simulink library "AEMS_Standard_Library"  (R2016b)
settings: Solver=ode45  StartTime=0.0  StopTime=10.0  RelTol=1e-3
undefined symbols (not defined in the file or in its folder): BkPY, carto, Cbx_extegr, Cbx_lpegrsys, Cbx_portegr, Cnx_bnk_nr_conf, Cnx_cyl_nr_conf, ConfigManagement, configuration_management, Cxx_dcm_io_tmr_end_xxxx, Cxx_dcm_rt_tmr_end, Cxx_DID_xxxx_IO_max, Cxx_DID_xxxx_IO_min, Cxx_egrhsofs, Cxx_vmaniegi, DEM_DEBOUNCE_FREEZE, DEM_DTR_CTL_INVISIBLE, DEM_DTR_CTL_NORMAL, Dem_DtrId2_XXX, Dem_DtrId3_XXX, Dem_DtrId4_XXX, Dem_DtrId5_XXX, Dem_DtrId6_XXX, Dem_DtrId7_XXX, Dem_DtrId8_XXX, Dem_DtrId9_XXX, Dem_DtrId_XXX, Dem_EnableConditionId2_XXX, Dem_EnableConditionId3_XXX, Dem_EnableConditionId4_XXX, Dem_EnableConditionId5_XXX, Dem_EnableConditionId6_XXX, Dem_EnableConditionId7_XXX, Dem_EnableConditionId8_XXX, Dem_EnableConditionId_XXX, Dem_EventId, Dem_EventId2_XXX, Dem_EventId3_XXX, Dem_EventId4_XXX, Dem_EventId5_XXX, Dem_EventId6_XXX, Dem_EventId7_XXX, Dem_EventId8_XXX, Dem_EventId9_XXX, Dem_EventId_Device_Faulttype, Dem_EventId_XXX, DEM_IUMPR_GENERAL_DENOMINATOR, DEM_OPCYC_IGNITION, Dem_RatioId2_XXX, Dem_RatioId3_XXX, Dem_RatioId4_XXX, Dem_RatioId5_XXX, Dem_RatioId6_XXX, Dem_RatioId7_XXX, Dem_RatioId8_XXX, Dem_RatioId_XXX, Dem_StorageConditionId2_XXX, Dem_StorageConditionId3_XXX, Dem_StorageConditionId4_XXX, Dem_StorageConditionId5_XXX ... (+65)
libraries: AEMS_Standard_Library x477, simulink x2
(part 9 of 39)

== system AEMS_Standard_Library/LOOKUP_TABLES ==
  AEMS_DIRECTLU_1D : Subsystem  Tag=[LIB]  mask(AEMS_DIRECTLU_1D){X=Variable, BkP=BreakPoint}
      mask prompts: X "Input Variable"; BkP "BreakPoint"
      mask help:
      | This block computes one dimensional interpolation based on the given Index and Ratio
      | Please document Variable & BreakPoint parameters
      |
      | Reference to AUTOSAR specification:
      |            - AUTOSAR Service Name:  Ifl_IpoCur_f32
      |            - Reference: SWS_Ifl_00021
      mask init:
      | numDims=1;
      | interpMethod=2;
      | bp1=[-5:0.5:5];
      | tableData=atan([-5:0.5:5]);
      | if strcmp(get_param(bdroot,'BlockDiagramType'),'library')
      |   dimsChar='n';
      | else
      |   dimsChar=sprintf('%d',numDims);
      | end
      | switch interpMethod
      |   case 1
      |     plottype = 'flatplot';
      |   case 2
      |     plottype = 'lineplot';
      |   otherwise
      |     plottype = 'splineplot';
      | end
      | [x,y,xaxes,yaxes]=ndlookico(plottype,numDims,'LookupNDInterp',tableData,bp1);
      settings: AttributesFormatString=%<MaskType>\nSource Variable : %<X>\nBreakPoint : %<BkP>
      mask Help:
      | eval('path_lib=fileparts(which(''AEMS_Standard_Library''));');
      | mskblk=get_param(gcbh,'MaskType');
      | doc_path = [path_lib '\help\',mskblk,'.pdf'];
      | eval('open(doc_path)');
      mask Display:
      | text(0.5,0.75,sprintf(' %s-D T(u)',dimsChar),'horizontalAlignment','center')
      | plot(x,y)
      | plot(xaxes,yaxes)
  AEMS_DIRECTLU_2D : Subsystem  Tag=[LIB]  mask(AEMS_DIRECTLU_2D){X=Variable_X, BkPX=BreakPoint_X, Y=Variable_Y, BkPY=BreakPoint_Y}
      mask prompts: X "Input Variable X"; BkPX "BreakPoint X"; Y "Input Variable Y"; BkPY "BreakPoint Y"
      mask help:
      | This block computes the 2D interpolation based on the given index and ratio
      | Please document Variable & BreakPoint parameters
      |
      | Reference to AUTOSAR specification:
      |           - AUTOSAR Service Name:  Ifl_IpoMap_f32
      |           - Reference: SWS_Ifl_00025
      mask init:
      | numDims=2;
      | interpMethod=2;
      | bp1=[1:10];
      | tableData=peaks(10);
      | if strcmp(get_param(bdroot,'BlockDiagramType'),'library')
      |   dimsChar='n';
      | else
      |   dimsChar=sprintf('%d',numDims);
      | end
      | switch interpMethod
      |   case 1
      |     plottype = 'flatplot';
      |   case 2
      |     plottype = 'lineplot';
      |   otherwise
      |     plottype = 'splineplot';
      | end
      | [x,y,xaxes,yaxes]=ndlookico(plottype,numDims,'LookupNDInterp',tableData,bp1);
      settings: AttributesFormatString=%<MaskType>\nSource X : %<X>\nBreakPoint X : %<BkPX>\nSource Y: %<Y>\nBreakPoint Y : %<BkPY>
      mask Help:
      | eval('path_lib=fileparts(which(''AEMS_Standard_Library''));');
      | mskblk=get_param(gcbh,'MaskType');
      | doc_path = [path_lib '\help\',mskblk,'.pdf'];
      | eval('open(doc_path)');
      mask Display:
      | text(0.50,0.90,sprintf(' %s-D T(u)',dimsChar),'horizontalAlignment','center')
      | plot(x,y)
      | plot(xaxes,yaxes)
  AEMS_DIRECTLU_INDEXED_1D : Subsystem  Tag=[LIB]  mask(AEMS_DIRECTLU_INDEXED_1D){X=Variable, BkP=BreakPoint}
      mask prompts: X "Input Quantity"; BkP "BreakPoint"
      mask help:
      | Indexed interpolation 1D using Index/Ration as input
      | Please documente Variable & BreakPoint parameters
      mask init:
      | numDims=1;
      | interpMethod=1;
      | bp1=[-5:0.5:5];
      | tableData=atan([-5:0.5:5]);
      | if strcmp(get_param(bdroot,'BlockDiagramType'),'library')
      |   dimsChar='n';
      | else
      |   dimsChar=sprintf('%d',numDims);
      | end
      | switch interpMethod
      |   case 1
      |     plottype = 'flatplot';
      |   case 2
      |     plottype = 'lineplot';
      |   otherwise
      |     plottype = 'splineplot';
      | end
      | [x,y,xaxes,yaxes]=ndlookico(plottype,numDims,'LookupNDInterp',tableData,bp1);
      settings: AttributesFormatString=%<MaskType>\nSource Variable : %<X>\nBreakPoint : %<BkP>
      mask Help:
      | eval('path_lib=fileparts(which(''AEMS_Standard_Library''));');
      | doc_path = [path_lib '\help\AEMS_DIRECTLU_INDEXED_1D.pdf'];
      | eval('open(doc_path)')
      mask Display:
      | text(0.5,0.75,sprintf(' %s-D T(u)',dimsChar),'horizontalAlignment','center')
      | plot(x,y)
      | plot(xaxes,yaxes)
  AEMS_DIRECTLU_INDEXED_2D : Subsystem  Tag=[LIB]  mask(AEMS_DIRECTLU_INDEXED_2D){X=Source_X, BkPX=BreakPoint_X, Y=Source_Y, BkPY=BreakPoint_Y}
      mask prompts: X "Input Quantity X"; BkPX "BreakPoint X"; Y "Input Quantity Y"; BkPY "BreakPoint Y"
      mask help:
      | Indexed interpolation 2D using Index/Ration as inputs
      | Please documente Variable & BreakPoint parameters
      mask init:
      | numDims=2;
      | interpMethod=1;
      | bp1=[1:10];
      | tableData=peaks(10);
      | if strcmp(get_param(bdroot,'BlockDiagramType'),'library')
      |   dimsChar='n';
      | else
      |   dimsChar=sprintf('%d',numDims);
      | end
      | switch interpMethod
      |   case 1
      |     plottype = 'flatplot';
      |   case 2
      |     plottype = 'lineplot';
      |   otherwise
      |     plottype = 'splineplot';
      | end
      | [x,y,xaxes,yaxes]=ndlookico(plottype,numDims,'LookupNDInterp',tableData,bp1);
      settings: AttributesFormatString=%<MaskType>\nSource X : %<X>\nBreakPoint X : %<BkPX>\nSource Y: %<Y>\nBreakPoint Y : %<BkPY>
      mask Help:
      | eval('path_lib=fileparts(which(''AEMS_Standard_Library''));');
      | doc_path = [path_lib '\help\AEMS_DIRECTLU_INDEXED_2D.pdf'];
      | eval('open(doc_path)')
      mask Display:
      | text(0.50,0.90,sprintf(' %s-D T(u)',dimsChar),'horizontalAlignment','center')
      | plot(x,y)
      | plot(xaxes,yaxes)
  AEMS_DYNAMIC_LUT_1D : Subsystem  Tag=[LIB]  mask(AEMS_DYNAMIC_LUT_1D){}
      mask help: This block executes an interpolation in a one-dimension cartography. The input variable is automatically limited by the breakpoint table dynamics.
      mask init:
      | numDims=1;
      | interpMethod=2;
      | if strcmp(get_param(bdroot,'BlockDiagramType'),'library')
      |   dimsChar='n';
      | else
      |   dimsChar=sprintf('%d',numDims);
      | end
      | switch interpMethod
      |   case 1
      |     plottype = 'flatplot';
      |   case 2
      |     plottype = 'lineplot';
      |   otherwise
      |     plottype = 'splineplot';
      | end
      settings: AttributesFormatString=%<MaskType>
      mask Help:
      | eval('path_lib=fileparts(which(''AEMS_Standard_Library''));');
      | doc_path = [path_lib '\help\AEMS_DYNAMIC_LUT_1D.pdf'];
      | eval('open(doc_path)')
      mask Display: disp('Dynamic\n\nInterp. (1D)\n')
  AEMS_INDEXED_LUT_1D : Subsystem  Tag=[LIB]  mask(AEMS_INDEXED_LUT_1D){map_x=Cxb, map_z=Cxd}
      mask prompts: map_x "Breakpoint table :"; map_z "Lookup table (1D) :"
      mask help: This block executes a research by indexing in an one-dimension cartography. The input variable is automatically limited by the breakpoint table dynamics.
      mask init:
      | numDims=1;
      | interpMethod=1;
      | bp1=double(map_x);
      | tableData=double(map_z);
      | if strcmp(get_param(bdroot,'BlockDiagramType'),'library')
      |   dimsChar='n';
      | else
      |   dimsChar=sprintf('%d',numDims);
      | end
      | switch interpMethod
      |   case 1
      |     plottype = 'flatplot';
      |   case 2
      |     plottype = 'lineplot';
      |   otherwise
      |     plottype = 'splineplot';
      | end
      | [x,y,xaxes,yaxes]=ndlookico(plottype,numDims,'LookupNDInterp',tableData,bp1);
      settings: AttributesFormatString=%<MaskType>\nBkPX=%<map_x>\nLUT=%<map_z>
      mask Help:
      | eval('path_lib=fileparts(which(''AEMS_Standard_Library''));');
      | doc_path = [path_lib '\help\AEMS_INDEXED_LUT_1D.pdf'];
      | eval('open(doc_path)')
      mask Display:
      | text(0.5,0.75,sprintf(' %s-D T(u)',dimsChar),'horizontalAlignment','center')
      | plot(x,y)
      | plot(xaxes,yaxes)
  AEMS_INDEXED_LUT_1D_TOL : Subsystem  Tag=[LIB]  mask(AEMS_INDEXED_LUT_1D_TOL){map_x=Cxb, map_z=Cxd, Tolerance=Cxx_Tol}
      mask prompts: map_x "Breakpoint table :"; map_z "Lookup table (1D) :"
      mask help:
      | This block executes an index in a one-dimension cartography with a tolerance applied to output values of decreasing transitions between adjacent breakpoint value zones. The input variables are automatically limited  by the breakpoint tables dynamics.
      |
      | To modify the Tolerance values, right-click on the block and select "Mask Parameters...".
      mask init: same as AEMS_Standard_Library/LOOKUP_TABLES/AEMS_INDEXED_LUT_1D
      settings: AttributesFormatString=%<MaskType>\nBkPX=%<map_x>\nLUT=%<map_z>\nTolerance=%<Tolerance>
      mask Help:
      | eval('path_lib=fileparts(which(''AEMS_Standard_Library''));');
      | doc_path = [path_lib '\help\AEMS_INDEXED_LUT_1D_TOL.pdf'];
      | eval('open(doc_path)')
      mask Display:
      | text(0.50,0.90,sprintf(' %s-D T(u) with tol.',dimsChar),'horizontalAlignment','center')
      | plot(x,y)
      | plot(xaxes,yaxes)
  AEMS_INDEXED_LUT_2D : Subsystem  Tag=[LIB]  mask(AEMS_INDEXED_LUT_2D){map_x=Cxb_x, map_y=Cxb_y, carto=Cxm}
      mask prompts: map_x "X Breakpoint table :"; map_y "Y Breakpoint table :"; carto "Lookup table (2D) :"
      mask help: This block executes an index in a two-dimension cartography. The input variables are automatically limited by the breakpoint tables dynamics.
      mask init:
      | numDims=2;
      | interpMethod=1;
      | bp1=double(map_x);
      | tableData=double(carto);
      | if strcmp(get_param(bdroot,'BlockDiagramType'),'library')
      |   dimsChar='n';
      | else
      |   dimsChar=sprintf('%d',numDims);
      | end
      | switch interpMethod
      |   case 1
      |     plottype = 'flatplot';
      |   case 2
      |     plottype = 'lineplot';
      |   otherwise
      |     plottype = 'splineplot';
      | end
      | [x,y,xaxes,yaxes]=ndlookico(plottype,numDims,'LookupNDInterp',tableData,bp1);
      settings: AttributesFormatString=%<MaskType>\nBkPX=%<map_x>\nBkPY=%<map_y>\nMAP=%<carto>
      mask Help:
      | eval('path_lib=fileparts(which(''AEMS_Standard_Library''));');
      | doc_path = [path_lib '\help\AEMS_INDEXED_LUT_2D.pdf'];
      | eval('open(doc_path)')
      mask Display:
      | text(0.50,0.90,sprintf(' %s-D T(u)',dimsChar),'horizontalAlignment','center')
      | plot(x,y)
      | plot(xaxes,yaxes)
  AEMS_INDEXED_LUT_2D_TOL : Subsystem  Tag=[LIB]  mask(AEMS_INDEXED_LUT_2D_TOL){map_x=Cxb_X, map_y=Cxb_Y, carto=Cxm, X_Tolerance=Cxx_Tol_X, Y_Tolerance=Cxx_Tol_Y}
      mask prompts: map_x "X Breakpoint table :"; map_y "Y Breakpoint table :"; carto "Lookup table (2D) :"
      mask help:
      | This block executes an index in a two-dimension cartography with a tolerance applied to output values of decreasing transitions between adjacent breakpoint value zones. The input variables are automatically limited  by the breakpoint tables dynamics.
      |
      | To modify the Tolerance values, right-click on the block and select "Mask Parameters...".
      mask init: same as AEMS_Standard_Library/LOOKUP_TABLES/AEMS_INDEXED_LUT_2D
      settings: AttributesFormatString=%<MaskType>\nBkPX=%<map_x>\nBkPY=%<map_y>\nMAP=%<carto>\nToleranceX=%<X_Tolerance>\nToleranceY=%<Y_Tolerance>
      mask Help:
      | eval('path_lib=fileparts(which(''AEMS_Standard_Library''));');
      | doc_path = [path_lib '\help\AEMS_INDEXED_LUT_2D_TOL.pdf'];
      | eval('open(doc_path)')
      mask Display:
      | text(0.50,0.90,sprintf(' %s-D T(u) with tol.',dimsChar),'horizontalAlignment','center')
      | plot(x,y)
      | plot(xaxes,yaxes)
  AEMS_INTERP : Subsystem  Tag=[LIB]  Description=This library calculates interpolation for 2 inputs.  mask(AEMS_INTERP){}
      mask help:
      | Interpolation for 2inputs
      |
      | output = input_of_ratio_1 * interpolate_ratio
      |          + input_of_ratio_0 * ( 1 - interpolate_ratio )
      |
      | I/O
      |     input_of_ratio_1
      |         Input of ratio term
      |     input_of_ratio_0
      |         Input of 1 - ratio term
      |     interpolate_ratio
      |         Interpolate Ratio ( 0 <= interpolate_ratio <= 1 )
      |
      |     output
      |         Output value
      settings: AttributesFormatString=%<MaskType>
      mask Help:
      | eval('path_lib=fileparts(which(''AEMS_Standard_Library''));');
      | mskblk=get_param(gcbh,'MaskType');
      | doc_path = [path_lib '\help\',mskblk,'.pdf'];
      | eval('open(doc_path)');
  AEMS_ITP3D : Subsystem  Tag=[LIB]  mask(AEMS_ITP3D){}
      mask help:
      | Vxx_fac is the parameter to interpolate between the three inputs
      |
      | The variable Vxx_fac is limited between 1 and 3.
      | If Vxx_fac == 1,  then Vxx_output == Vxx_in1
      | If Vxx_fac == 2,  then Vxx_output == Vxx_in2
      | If Vxx_fac == 3 , then Vxx_output == Vxx_in3
      |
      | If the Vxx_fac is not an integer, then Vxx_out is the result of interpolation.
      settings: AttributesFormatString=%<MaskType>
      mask Help:
      | eval('path_lib=fileparts(which(''AEMS_Standard_Library''));');
      | doc_path = [path_lib '\help\AEMS_ITP3D.pdf'];
      | eval('open(doc_path)')
      mask Display: disp('AEMS_ITP3D');
  AEMS_LUT_1D : Subsystem  Tag=[LIB]  mask(AEMS_LUT_1D){map_x=Cxb, map_z=Cxp}
      mask prompts: map_x "Breakpoint array :"; map_z "Lookup table (1D) :"
      mask help:
      | This block executes an interpolation in one-dimensional cartography. The input variable is automatically limited  by the breakpoint table dynamics.
      |
      | Reference to AUTOSAR specification:
      |            - AUTOSAR Service Name:  Ifl_IntIpoCur_f32_f32
      |            - Reference: SWS_Ifl_00035
      mask init:
      | numDims=1;
      | interpMethod=2;
      | bp1=double(map_x);
      | tableData=double(map_z);
      | if strcmp(get_param(bdroot,'BlockDiagramType'),'library')
      |   dimsChar='n';
      | else
      |   dimsChar=sprintf('%d',numDims);
      | end
      | switch interpMethod
      |   case 1
      |     plottype = 'flatplot';
      |   case 2
      |     plottype = 'lineplot';
      |   otherwise
      |     plottype = 'splineplot';
      | end
      | [x,y,xaxes,yaxes]=ndlookico(plottype,numDims,'LookupNDInterp',tableData,bp1);
      settings: AttributesFormatString=%<MaskType>\nBkPX=%<map_x>\nLUT=%<map_z>
      mask Help:
      | eval('path_lib=fileparts(which(''AEMS_Standard_Library''));');
      | mskblk=get_param(gcbh,'MaskType');
      | doc_path = [path_lib '\help\',mskblk,'.pdf'];
      | eval('open(doc_path)');
      mask Display:
      | text(0.5,0.75,sprintf(' %s-D T(u)',dimsChar),'horizontalAlignment','center')
      | plot(x,y)
      | plot(xaxes,yaxes)
  AEMS_LUT_2D : Subsystem  Tag=[LIB]  mask(AEMS_LUT_2D){map_x=Cxb_x, map_y=Cxb_y, carto=Cxm}
      mask prompts: map_x "X Breakpoint array :"; map_y "Y Breakpoint array :"; carto "Lookup table (2D) :"
      mask help:
      | This block executes an interpolation in two-dimensional cartography. The input variables are automatically limited  by the breakpoint tables dynamics.
      |
      | Reference to AUTOSAR specification:
      |            - AUTOSAR Service Name:  Ifl_IntIpoMap_f32f32_f32
      |            - Reference: SWS_Ifl_00041
      mask init:
      | numDims=2;
      | interpMethod=2;
      | bp1=double(map_x);
      | tableData=double(carto);
      | if strcmp(get_param(bdroot,'BlockDiagramType'),'library')
      |   dimsChar='n';
      | else
      |   dimsChar=sprintf('%d',numDims);
      | end
      | switch interpMethod
      |   case 1
      |     plottype = 'flatplot';
      |   case 2
      |     plottype = 'lineplot';
      |   otherwise
      |     plottype = 'splineplot';
      | end
      | [x,y,xaxes,yaxes]=ndlookico(plottype,numDims,'LookupNDInterp',tableData,bp1);
      settings: AttributesFormatString=%<MaskType>\nBkPX=%<map_x>\nBkPY=%<map_y>\nMAP=%<carto>
      mask Help:
      | eval('path_lib=fileparts(which(''AEMS_Standard_Library''));');
      | mskblk=get_param(gcbh,'MaskType');
      | doc_path = [path_lib '\help\',mskblk,'.pdf'];
      | eval('open(doc_path)');
      mask Display:
      | text(0.50,0.90,sprintf(' %s-D T(u)',dimsChar),'horizontalAlignment','center')
      | plot(x,y)
      | plot(xaxes,yaxes)
  AEMS_PRE_INTERP : Subsystem  Tag=[LIB]  mask(AEMS_PRE_INTERP){Cxb=Breakpoint}
      mask prompts: Cxb "BreakPoint array"
      mask help:
      | The block computes the Index and Ratio of input variable in a breakpoint data
      |
      | Reference to AUTOSAR specification:
      |            - AUTOSAR Service Name:  Ifl_DPSearch_f32
      |            - Reference: SWS_Ifl_00010
      mask init:
      | fig='f';
      | f='f';
      | [x,y]=ndlookico('bpplotdata',fig);
      | [xp,yp]=ndlookico('bppatchdata');
      settings: AttributesFormatString=%<MaskType>\nBKPT = %<Cxb>
      mask Help:
      | eval('path_lib=fileparts(which(''AEMS_Standard_Library''));');
      | mskblk=get_param(gcbh,'MaskType');
      | doc_path = [path_lib '\help\',mskblk,'.pdf'];
      | eval('open(doc_path)');
      mask Display:
      | text(2.3*0.13, .95*0.85, '','HorizontalAlignment','center','VerticalAlignment','middle');
      | text(0.4, 0.53, '','HorizontalAlignment','center','VerticalAlignment','base');
      | text(0.88, 0.3, '','HorizontalAlignment','center','VerticalAlignment','middle');
      | plot(0.3+0.4*x,0.4+0.3*y);
      | patch(0.3+0.4*xp, 0.4+0.3*yp);

== system AEMS_Standard_Library/MATH ==
  AEMS_CLAMP : Subsystem  Tag=[LIB]  mask(AEMS_CLAMP){}
      mask help:
      | This block returns the bounded value (Output), determined according to the following equation
      |
      | Output = Min, if Input ≤ Min
      | Output = Max, if Input ≥ Max
      | Output = Input, if Min < val < Max
      |
      | Reference to AUTOSAR specification:
      |          - AUTOSAR Service Name:  Mfl_Limit_f32
      |          - Reference: SWS_Mfl_00122
      settings: AttributesFormatString=%<MaskType>
      mask Help:
      | eval('path_lib=fileparts(which(''AEMS_Standard_Library''));');
      | mskblk=get_param(gcbh,'MaskType');
      | doc_path = [path_lib '\help\',mskblk,'.pdf'];
      | eval('open(doc_path)');
      mask Display: plot([0.2 0.8],[0.5 0.5],[0.5 0.5],[0.2 0.8],[0.2 0.35 0.65 0.8],[0.2 0.2 0.8 0.8])
  AEMS_DIVISION_BY_ZERO : Subsystem  Tag=[LIB]  mask(AEMS_DIVISION_BY_ZERO){Tolerence=1.1920929e-07}
      mask prompts: Tolerence "Denominator Tolerance"
      mask help:
      | This block outputs the value of the division operation "num / den ". If the "den" is exactly 0,the output will be the value at the port "ans_of_0div"
      |
      | In order to avoid "Inf" at output ,"den" must not take values close to zero.
      | Please provide Denominator tolerance(lowest possible resolution that denominator can take) in the mask.
      | Default tolerance: 1.1920929e-07
      mask init:
      | if Tolerence < 0
      |     errordlg('Denominator Tolerance value must be positive', 'Error Message');
      | end
      settings: AttributesFormatString=%<MaskType>\nDenominator Tolerance = %<Tolerence>
      mask Help:
      | eval('path_lib=fileparts(which(''AEMS_Standard_Library''));');
      | doc_path = [path_lib '\help\AEMS_DIVISION_BY_ZERO.pdf'];
      | eval('open(doc_path)')
      mask Display:
      | port_label('input',1,'den')
      | port_label('input',2,'num')
      | port_label('output',1,'result')
      | port_label('input',3,'ans_of_0div')
      | disp('Division \n no division by "0"')
      | 
      | disp('\n\n\n\n!! This Block is obsolete and should be replaced \n by AEMS_PROTECTED_DIVISION instead')
  AEMS_EXTRACT_INDEX : Subsystem  Tag=[LIB]  mask(AEMS_EXTRACT_INDEX){}
      mask help:
      | This block is built to extract the previous value (Previous_Value) and the corresponding index (Index_prev) as well as the next value (Next_Value) and its corresponding index (Index_nxt) of an increasing vector when compared to a scalar input (X).
      |
      | If the scalar input is smaller than all elements of Vector. The previous index is the smallest index, the next index is equal to previous index plus 1.
      |
      | If the scalar input is greater than all elements of Vector, the previous value and the next value are the same; it is the last value of the vector. The previous index and the next have the greatest index.
      settings: AttributesFormatString=%<MaskType>
      mask Help:
      | eval('path_lib=fileparts(which(''AEMS_Standard_Library''));');
      | doc_path = [path_lib '\help\AEMS_EXTRACT_INDEX.pdf'];
      | eval('open(doc_path)')
  AEMS_IGN_TO_PHY : Subsystem  Tag=[LIB]  mask(AEMS_IGN_TO_PHY){nb_cyl_max=6}
      mask prompts: nb_cyl_max "Limitation of number of cylinders"
      mask help:
      | Converts a vector that is supposed to be an ignition order into cylinder physical order given by the "order vector" calibration input.
      | Number of cylinders can be handled is from 1 cylinder to 6 cylinders. Calibration should indicate 0 when cylinders are not used.
      | Limitation of number of cylinders : the number of cylinders really used in input/output.
      | If some elements of the vectors are not used, a replacement value is asked as an input of the block.
      |
      | -INPUTS-
      | Order_vector: Order to sort
      | Replacement value: Value to be replaced for unused index
      | Ignition order:Physical order: Vector to be sorted
      |
      | -OUTPUTS-
      | Physical order: Ouput vector sorted
      |
      | -PARAMETERS-
      | Limitation of number of cylinders: Limit of cylinder number
      mask init:
      | Input='Ignition order';
      | Output='Physical order';
      settings: AttributesFormatString=%<MaskType>\nLimitation of number of cylinders = %<nb_cyl_max>
      mask Help:
      | eval('path_lib=fileparts(which(''AEMS_Standard_Library''));');
      | doc_path = [path_lib '\help\AEMS_IGN_TO_PHY.pdf'];
      | eval('open(doc_path)')
      mask Display:
      | port_label('input',1,'Order vector');
      | port_label('input',2,'Replacement value');
      | port_label('input',3,Input);
      | port_label('output',1,Output);
  AEMS_MATRIX_INVERSION : Subsystem  Tag=[LIB]  mask(AEMS_MATRIX_INVERSION){}
      mask help:
      | Computes the inversion of a 3*3 matrix.
      |
      | Input: Must be a 3*3 matrix.
      | Output: Inverse of the given input 3*3 matrix.
      |
      | For Example, If Matrix A (3*3 dimension), then the inverse is computed by, Inverse A = (1/Det(A)*Adj(A)).
      |
      | Note: If the Det(A) =0, then matrix inversion is not possible.
      | So, the output will be the alternate input.
      settings: AttributesFormatString=%<MaskType>
      mask Help:
      | eval('path_lib=fileparts(which(''AEMS_Standard_Library''));');
      | doc_path = [path_lib '\help\AEMS_MATRIX_INVERSION.pdf'];
      | eval('open(doc_path)')
      mask Display:
      | disp('\n\n\n\n\n\nAEMS_MATRIX_INVERSION')
      | plot([0.32 0.32],[0.3 0.9],[0.62 0.62],[0.3 0.9])
      | text(0.35,0.8,'x1');
      | text(0.45,0.8,'x2');
      | text(0.55,0.8,'x3');
      | text(0.35,0.6,'y1');
      | text(0.45,0.6,'y2');
      | text(0.55,0.6,'y3');
      | text(0.35,0.4,'z1');
      | text(0.45,0.4,'z2');
      | text(0.55,0.4,'z3');
      | plot([0.32 0.35],[0.3 0.3])
      | plot([0.59 0.62],[0.3 0.3])
      | plot([0.32 0.35],[0.9 0.9])
      | plot([0.59 0.62],[0.9 0.9])
      | plot([0.65 0.67],[0.92 0.92])
      | %plot([0.70 0.70],[0.85 1])
      | text(0.68,0.9,'1')
  AEMS_PHY_TO_IGN : Subsystem  Tag=[LIB]  mask(AEMS_PHY_TO_IGN){nb_cyl_max=6}
      mask prompts: nb_cyl_max "Limitation of number of cylinders"
      mask help:
      | Converts a vector that is supposed to be in Cylinder Physical order to an ignition order given by the "Order vector" calibration input (always of dimension 1x6).
      | Number of cylindres can be handled is from 1 cylinder to 6 cylinders.
      | Calibration should indicate 0 when cylinders are not used.
      |
      | Limitation of number of cylinders : the number of cylinders really used in input/output.
      |
      | If some elements of the vectors are not used, a replacement value is asked as an input of the block.
      mask init:
      | Output='Ignition order';
      | Input='Physical order';
      settings: AttributesFormatString=%<MaskType>\nLimitation of number of cylinders = %<nb_cyl_max>
      mask Help:
      | eval('path_lib=fileparts(which(''AEMS_Standard_Library''));');
      | doc_path = [path_lib '\help\AEMS_PHY_TO_IGN.pdf'];
      | eval('open(doc_path)')
      mask Display:
      | port_label('input',1,'Order vector');
      | port_label('input',2,'Replacement value');
      | port_label('input',3,Input);
      | port_label('output',1,Output);
  AEMS_PROTECTED_DIVISION : Subsystem  Tag=[LIB]  mask(AEMS_PROTECTED_DIVISION){out_mode=Numerator / Tolerance -> Output, tolerance=0.01}
      mask prompts: out_mode "Output when |Denominator| < Tolerance"; tolerance "Denominator Tolerance"
      mask help:
      | This block outputs the value of the division operation "num / den".
      | When the "den" is less than "Denominator Tolerance", then there are two possible outputs that can be chosen:
      | Case 1: The output will be the value at the port "default_output".
      | Case 2: The output will be "Numerator/Tolerance".
      |
      | Note :
      | For TargetLink Code generation, "protect against division by zero in production code" property should be disabled for the divide block present inside this Library.
      |
      | The "tolerance" value has to be given in accordance with the "den" (denominator) datatype.
      mask init:
      | This_Blk=gcb;
      | if tolerance < 0
      |     errordlg('Denominator tolerance value must be positive', 'Error Message');
      | end
      | 
      | ports = get_param(gcb,'PortHandles');
      | nbinport = length(ports.Inport);
      | 
      | if(out_mode == 1) %default ouput, three inputs
      |     if(nbinport==2)%change things => three inputs
      |     delete_line(This_Blk,'Divide/1','result/1');
      |     add_block('built-in/Inport',[This_Blk,'/default_output'],'Position',[85   448   105   462],'BackgroundColor','Green');
      |     add_block('simulink/Signal Routing/Switch',[This_Blk,'/Switch1'],'Position',[695   293   735   487],'Criteria','u2 ~= 0',...
      |          'AttributesFormatString','Criteria=%<Criteria>','ShowName','off');
      |     add_line(This_Blk,'Divide/1','Switch1/1','autorouting','on');
      |     add_line(This_Blk,'RelationalOperator/1','Switch1/2','autorouting','on');
      |     add_line(This_Blk,'default_output/1','Switch1/3','autorouting','on');
      |     add_line(This_Blk,'Switch1/1','result/1','autorouting','on');
      |     end
      |     ModeStr = 'Default_Output -> Output';
      |     
      | elseif(out_mode == 2) % tol used as denominator, two inputs
      |     if(nbinport==3)%change things => two inputs
      |     delete_block([This_Blk,'/default_output']);
      |     delete_block([This_Blk,'/Switch1']);
      |     delete_line(find_system(This_Blk,'FindAll','on','FollowLinks','on','LookUnderMasks','on','Type','line','Connected','off')); 
      |     add_line(This_Blk,'Divide/1','result/1');
      |     end
      |     ModeStr = 'Numerator / Tolerance -> Output';
      | end
      settings: AttributesFormatString=%<MaskType>\nOutput when |Denominator| < Tolerance = %<out_mode>\nDenominator Tolerance = %<tolerance>
      mask Help:
      | eval('path_lib=fileparts(which(''AEMS_Standard_Library''));');
      | mskblk=get_param(gcbh,'MaskType');
      | doc_path = [path_lib '\help\',mskblk,'.pdf'];
      | eval('open(doc_path)');
      mask TypeOptions out_mode: Default_Output -> Output | Numerator / Tolerance -> Output
      mask Display: disp(['Protected division\n' ModeStr])
  AEMS_SORT : Subsystem  Tag=[LIB]  TreatAsAtomicUnit=on  mask(AEMS_SORT){N=20, SortChoice=Ascendant Median, IndexSelection=on}
      mask prompts: N "Number of input element"; SortChoice "Way of sorting"; IndexSelection "Selectable Index"
      mask help:
      | This block is used to sort one-dimensional arrays and to get the median in the case of the ascending sorting.
      |
      | You have the choice between 3 options which are :
      | - Option 1 : Sort in ascending order
      | - Option 2 : Sort in descending order
      | - Option 3 : Sort in ascending order and get the corresponding median
      |
      | In addition, you can choose or not to select the number of element that you want to sort in your table and get the median number with the Option 3. (This input number N is the desired size of the input matrix that you want to sort, from 0 to N index ).
      |
      | - INPUTS -
      |
      | If the "selectable index" option is checked
      | - Disordered 1-D vector
      | - The first N numbers that you want to sort (zero-based index)
      |
      | If the "selectable index" option is unchecked :
      | - Disordered 1-D vector
      |
      | - OUTPUTS -
      |
      | =>For the Option 1&2
      | - If the check box "selectable index" is checked : Sorted vector of the first N numbers
      | - If the checkbox "selectable index" is not checked : Sorted vector of  the whole matrix
      |
      | =>For the Option 3
      | - If the checkbox "selectable index" is checked : Sorted vector and median of the first N numbers
      | - If the checkbox "selectable index" is not checked : Sorted vector and median of  the whole matrix
      |
      | NOTE: The maximum value allowed for the input "Selectable index" is 127.
      mask init:
      | block = find_system(gcb,...
      |           'LookUnderMasks','on',...
      |           'FollowLinks','on','Name','Median_Out');
      | 
      | %%%%%%%%%%%%%%
      | 
      | %condition for the selectable index
      | 
      | if strcmpi(IndexSelection,'on')
      |     
      |     if ismember(get_param([gcb, '/Index'],'BlockType'),{'Inport'})   
      |     else
      |      replace_block(gcb,'FollowLinks','on','Name','Index','built-in/Inport','noprompt');
      |      set_param([gcb, '/Index'],'BackgroundColor','green')
      |     end
      | 
      | else
      |    replace_block(gcb,'FollowLinks','on','Name','Index','Constant','noprompt');
      |    set_param([gcb, '/Index'], 'Value', 'N-1','OutDataTypeStr','uint8');
      | end
      | 
      | %%%%%%%%%%%%%%
      | 
      | set_param([gcb, '/For_loop_1/For_loop_2/Comparison/Selector'], 'InputPortWidth', 'N')
      | set_param([gcb, '/For_loop_1/For_loop_2/Comparison/Selector1'], 'InputPortWidth', 'N')
      | set_param([gcb, '/For_loop_1/For_loop_2/UnitDelay'], 'InitialCondition', 'zeros(1,N)')
      | 
      | switch SortChoice
      |     case 1
      |         set_param([gcb,'/For_loop_1/For_loop_2/Comparison/Relational_Operator'], 'Operator', '>')
      |         if ~isempty(block)
      |             delete_line([gcb],'For_loop_1/1','AEMS_SORT_MEDIAN/1')
      |             delete_line([gcb],'Index/1','AEMS_SORT_MEDIAN/2')
      |             delete_line([gcb],'AEMS_SORT_MEDIAN/1','Median_Out/1')
      |             delete_block([gcb,'/AEMS_SORT_MEDIAN'])
      |             delete_block(block);
      |         end
      |             
      |             
      |     case 2
      |         set_param([gcb, '/For_loop_1/For_loop_2/Comparison/Relational_Operator'], 'Operator', '<')
      |         if ~isempty(block)
      |             delete_line([gcb],'For_loop_1/1','AEMS_SORT_MEDIAN/1')
      |             delete_line([gcb],'Index/1','AEMS_SORT_MEDIAN/2')
      |             delete_line([gcb],'AEMS_SORT_MEDIAN/1','Median_Out/1')
      |             delete_block([gcb,'/AEMS_SORT_MEDIAN'])
      |             delete_block(block);
      |         end
      |             
      | 
      |     case 3 
      |         set_param([gcb, '/For_loop_1/For_loop_2/Comparison/Relational_Operator'], 'Operator', '>')
      |         if isempty(block)
      |             add_block('built-in/Outport',[gcb,'/Median_Out'],'Position',[815 178 845 192],'BackgroundColor','Orange');
      |             add_block('AEMS_Standard_Library/SUB/AEMS_SORT_MEDIAN',[gcb,'/AEMS_SORT_MEDIAN'],'Position',[525 139 720 226]);
      |             add_line([gcb],{'For_loop_1/1','Index/1'},{'AEMS_SORT_MEDIAN/1','AEMS_SORT_MEDIAN/2'},'autorouting','on')
      |             add_line([gcb],'AEMS_SORT_MEDIAN/1','Median_Out/1','autorouting','on')
      |         end
      |  end
      settings: AttributesFormatString=%<MaskType>\nSize of input vector : %<N>\n Sort : %<SortChoice>\nSelectable Index = %<IndexSelection>
      mask Help:
      | eval('path_lib=fileparts(which(''AEMS_Standard_Library''));');
      | doc_path = [path_lib '\help\AEMS_SORT.pdf'];
      | eval('open(doc_path)')
      mask TypeOptions SortChoice: Ascendant | Descendant | Ascendant Median
      mask Display:
      | set_param(gcb,'BackgroundColor','yellow');
      | 
      | text(0.40,0.1,'AEMS_SORT');
      | 
      | %upper box
      | plot([0.3 0.35],[0.7 0.7], [0.3 0.35],[0.65 0.65], [0.3 0.3],[0.7 0.65], [0.35 0.35],[0.7 0.65])
      | plot([0.4 0.45],[0.7 0.7], [0.4 0.45],[0.65 0.65], [0.4 0.4],[0.7 0.65], [0.45 0.45],[0.7 0.65])
      | plot([0.5 0.55],[0.7 0.7], [0.5 0.55],[0.65 0.65], [0.5 0.5],[0.7 0.65], [0.55 0.55],[0.7 0.65])
      | plot([0.6 0.65],[0.7 0.7], [0.6 0.65],[0.65 0.65], [0.6 0.6],[0.7 0.65], [0.65 0.65],[0.7 0.65])
      | 
      | %lower box
      | plot([0.3 0.35],[0.35 0.35], [0.3 0.35],[0.3 0.3], [0.3 0.3],[0.3 0.35], [0.35 0.35],[0.3 0.35])
      | plot([0.4 0.45],[0.35 0.35], [0.4 0.45],[0.3 0.3], [0.4 0.4],[0.3 0.35], [0.45 0.45],[0.3 0.35])
      | 
      | %boxes
      | plot([0.5 0.55],[0.35 0.35], [0.5 0.55],[0.3 0.3], [0.5 0.5],[0.3 0.35], [0.55 0.55],[0.3 0.35])
      | plot([0.6 0.65],[0.35 0.35], [0.6 0.65],[0.3 0.3], [0.6 0.6],[0.3 0.35], [0.65 0.65],[0.3 0.35])
      | 
      | %lines
      | plot([0.32 0.62],[0.65 0.35], [0.62 0.42],[0.65 0.35], [0.42 0.32],[0.65 0.35], [0.52 0.52],[0.65 0.35])
      | 
      | %arrows
      | plot([0.32 0.32],[0.35 0.43], [0.32 0.36],[0.35 0.39])
      | plot([0.42 0.44],[0.35 0.43], [0.42 0.465],[0.35 0.37])
      | plot([0.52 0.5],[0.35 0.41], [0.52 0.54],[0.35 0.4])
      | plot([0.62 0.6],[0.35 0.4], [0.62 0.58],[0.35 0.36])
      | 
      | port_label('input',1,'Vector to sort');
      | 
      | port_label('output',1,'Sorted vector 0:N');
      | 
      | switch SortChoice
      | 
      |     case 3
      |         port_label('output',2,'Median vector 0:N');
      | end
      | 
      | 
      | if strcmpi(IndexSelection,'on')
      |     port_label('input',2,'Selectable index 0:N');
      | end
  AEMS_SQRT : Subsystem  Tag=[LIB]  mask(AEMS_SQRT){FunctionOfSqrt=signedSqrt}
      mask prompts: FunctionOfSqrt "Function of Sqrt"
      mask help:
      | This block returns the square root of the input. (signedSqrt / rSqrt)
      | It can perform square root operation for both signed and unsigned values. But according to AUTOSAR service Mfl_Sqrt_f32 only unsigned inputs are allowed.
      |
      | Reference to AUTOSAR specification:
      | - AUTOSAR Service Name:  Mfl_Sqrt_f32 (Ref. [SWS_Mfl_00135])
      |
      | Function of Sqrt:
      | <signedSqrt>: Square root of the absolute value of the input, multiplied by the sign of the input
      | <rSqrt>: Reciprocal of square root of the input
      mask init:
      | This_Blk=gcb;
      | Bpath = [This_Blk,'/Sqrt'];
      | FunctionOfSqrt = get_param(This_Blk,'FunctionOfSqrt');
      | set_param(Bpath,'Operator',FunctionOfSqrt);
      settings: AttributesFormatString=|
      | %<MaskType> \n Service name : Mfl_Sqrt_f32
      | Function of Sqrt  : %<FunctionOfSqrt>
      mask Help:
      | eval('path_lib=fileparts(which(''AEMS_Standard_Library''));');
      | mskblk=get_param(gcbh,'MaskType');
      | doc_path = [path_lib '\Help\',mskblk,'.pdf'];
      | eval('open(doc_path)');
      mask TypeOptions FunctionOfSqrt: signedSqrt | rSqrt
      mask Display: disp('AEMS_SQRT\n');

== system AEMS_Standard_Library/MEM ==
  AEMS_NVM_SET : UnitDelay  Tag=[LIB]  InitialCondition=initial_value  SampleTime=-1  mask(AEMS_NVM_SET){initial_value=0}
      mask help: 'Unit Delay' for NVM(non volatile memory).
      settings: AttributesFormatString=<initial=%<initial_value>>
      mask Display:
      | % patch([0 100 100 0], [100 100 0 0], [1 1 1])
      | 
      | text(50,50,'\fontsize{14}1/Z','HorizontalAlignment','center',...
      |     'VerticalAlignment','middle','texmode','on')
      | text(92,100,'\fontsize{10}NVM ','HorizontalAlignment','right',...
      |     'VerticalAlignment','top','texmode','on')
      | 
      | plot([0,100],[0,0])
      | plot([0,100],[100,100])
      | plot([0,0],[0,100])
      | plot([100,100],[0,100])
  AEMS_NVM_WRITEONFLY : Subsystem  Tag=[LIB]  mask(AEMS_NVM_WRITEONFLY){NumInputs=1, ChId=<AEMS_Specification_Name>, TriggerType=Rising edge}
      mask prompts: NumInputs "Number of Inputs"; ChId "Channel Name (AEMS Specification Name):"; TriggerType "Trigger Type"
      mask help:
      | This block allows to represent the NVM write ON FLY Storage Type which will generate during codegeneration process (example):
      |
      | if (NVM_trigger && !NVMtrigger_old )
      |        Event_WriteOnFly_<AEMS_Specification_Name>();
      | end
      |
      | The parameter TriggerType can either be Rising edge (default) or Enable.
      |
      | NOTE: Input must not be zero.
      mask init:
      | % AEMSPattern='^[a,b]_...._...._..._\w*';
      | % if isempty(regexp(ChId,AEMSPattern,'once'))
      | %    errordlg('Error! Channel name is not correct');
      | % end
      | ThisBlk=gcb;
      | BlkType_Of_TriggerType  = get_param([ThisBlk '/PortType'] ,'BlockType');
      | TriggerType=get_param(ThisBlk,'TriggerType');
      | if isequal(TriggerType,'Rising edge')
      |     if strcmp(BlkType_Of_TriggerType ,'TriggerPort')
      |     %do nothing
      |     else
      |     replace_block(ThisBlk,'FollowLinks','on','Name','PortType','simulink/Ports & Subsystems/Trigger','noprompt');
      |     end
      | else
      |     if strcmp(BlkType_Of_TriggerType ,'EnablePort')
      |     %do nothing
      |     else
      |     replace_block(ThisBlk,'FollowLinks','on','Name','PortType','simulink/Ports & Subsystems/Enable','noprompt');
      |     end
      | end
      | set_param([ThisBlk '/PortType'],'AttributesFormatString','StatesWhenEnabling = %<StatesWhenEnabling>');
      | 
      | N_Inports=str2num(get_param(ThisBlk,'NumInputs'));
      | if isequal(N_Inports,0)
      |     errordlg('Error!! Input must not be 0');
      |     set_param(ThisBlk,'NumInputs','');
      | else
      |     a = 150;
      |     Old_inports = find_system(ThisBlk,'SearchDepth',1,'LookUnderMasks','on','FollowLinks','on','BlockType','Inport');
      |     if N_Inports ~= (length(Old_inports))
      |         incount=0;
      |         for i=1:length(Old_inports)
      |             hanblk=get_param(Old_inports{i},'handle');
      |             %         if ~strcmpi(get_param(hanblk,'Name'),'Vbx_enable')
      |             incount=incount+1;
      |             blkDet=get(hanblk);
      |             pos=blkDet.PortConnectivity(1).Position;
      |             try
      |                 delete_line(ThisBlk,pos);
      |                 delete_block([ThisBlk '/In' num2str(incount)]);
      |                 delete_block([ThisBlk '/Terminator' num2str(incount)]);
      |             end
      |             %         end
      |         end
      |         for i=1:N_Inports
      |             b = i*50;
      |             try
      |                 add_block('built-in/Inport',[ThisBlk '/In' num2str(i)],'Position',[a-60 b-5 a-40 b+8],'BackgroundColor','green');
      |                 add_block('built-in/Terminator',[ThisBlk '/Terminator' num2str(i)],'Position',[a-5 b-5 a+10 b+8],'Showname','off');
      |                 add_line(ThisBlk,['In' num2str(i) '/1'],['Terminator' num2str(i) '/1' ],'Autorouting','On');
      |             end
      |         end
      |     end
      | end
      settings: RTWSystemCode=Inline
      settings: AttributesFormatString=|
      | %<MaskType>
      | Number of Inputs = %<NumInputs>
      | Channel Name: %<ChId>
      | Trigger Type: %<TriggerType>
      mask Help:
      | eval('path_lib=fileparts(which(''AEMS_Standard_Library''));');
      | mskblk=get_param(gcbh,'MaskType');
      | doc_path = [path_lib '\help\',mskblk,'.pdf'];
      | eval('open(doc_path)');
      mask TypeOptions TriggerType: Rising edge | Enable
      mask Display: disp('AEMS_NVM_WRITEONFLY');
  AEMS_NVM_WRITEONFLY_ENABLE : Subsystem  Tag=[LIB]  mask(AEMS_NVM_WRITEONFLY_ENABLE){ChId=<AEMS_Specification_Name>}
      mask prompts: ChId "Channel Name (AEMS Specification Name):"
      mask help:
      | This block allows to represent the NVM write ON FLY Storage Type which will generate during codegeneration process (example):
      |
      | if (NVM_trigger && !NVMtrigger_old )
      |        Event_WriteOnFly_<AEMS_Specification_Name>();
      | end
      settings: RTWSystemCode=Inline
      settings: AttributesFormatString=|
      | %<MaskType>
      | Channel Name: %<ChId>
      mask Help:
      | eval('path_lib=fileparts(which(''AEMS_Standard_Library''));');
      | mskblk=get_param(gcbh,'MaskType');
      | doc_path = [path_lib '\help\',mskblk,'.pdf'];
      | eval('open(doc_path)');
      mask Display:
      | disp('AEMS_NVM_WRITEONFLY_ENABLE');
      | disp('\n\n\n\n This Block is obsolete!! \n Use AEMS_NVM_WRITEONFLY instead');

== system AEMS_Standard_Library/SAFETY ==
  AEMS_FSL_RAM_ASIL_TO_QM : DataTypeConversion  Tag=[LIB]  SaturateOnIntegerOverflow=on  mask(AEMS_FSL_RAM_ASIL_TO_QM){}
      mask help:
      | Copy RAM from ASIL area to QM area
      |
      | I/O
      |  input
      |    Parameter in ASIL area to be copied in QM area.
      |
      |  output
      |    Parameter in QM area copied from ASIL area.
      settings: AttributesFormatString=%<MaskType>
      mask Help:
      | eval('path_lib=fileparts(which(''AEMS_Standard_Library''));');
      | doc_path = [path_lib '\help\AEMS_FSL_RAM_ASIL_TO_QM.pdf'];
      | eval('open(doc_path)')
      mask Display: disp('RAM copy from ASIL to QM')
  AEMS_FSL_RAM_QM_TO_ASIL : DataTypeConversion  Tag=[LIB]  SaturateOnIntegerOverflow=on  mask(AEMS_FSL_RAM_QM_TO_ASIL){}
      mask help:
      | Copy RAM from QM area to ASIL area
      |
      | I/O
      |  input
      |    Parameter in QM area to be copied in ASIL area.
      |
      |  output
      |    Parameter in ASIL area copied from QM area.
      settings: AttributesFormatString=%<MaskType>
      mask Help:
      | eval('path_lib=fileparts(which(''AEMS_Standard_Library''));');
      | doc_path = [path_lib '\help\AEMS_FSL_RAM_QM_TO_ASIL.pdf'];
      | eval('open(doc_path)');
      mask Display: disp('RAM copy from QM to ASIL')
  AEMS_SAFETY_AND_REGULATION : Subsystem  mask(AEMS_SAFETY_AND_REGULATION){security=on, regulation=on}
      mask prompts: security "Security characteristics"; regulation "Regulatory characteristics"
      mask help: To insure traceability of Safety and Regulation requirements
      mask Display:
      | th = 0:pi/20:2*pi;
      | crc = [0.45 * cos(th) + 0.5; 0.45 * sin(th) + 0.5];
      | plot(crc(1,:),crc(2,:))
      | 
      | plot([0.5 0.87 0.13 0.5],[0.05 0.75 0.75 0.05]);
      | 
      | if security ~= 0
      |     text(0.87,0.8, 'S');
      |     if security > 1
      |         text(0.05,0.8, int2str(security));
      |     end
      | end
      | 
      | 
      | if regulation ~= 0
      |     text(0.87,0.2, 'R');
      |     if regulation > 1
      |         text(0.05,0.2, int2str(regulation));
      |     end
      | end
